simulink model "WECModel"  (R2021a)
settings: Solver=VariableStepAuto  StartTime=0.0  StopTime=30  RelTol=1e-3
undefined symbols (not defined in the file): A_c, alpha, beta, c33, delta, f_excitation_imaginary, f_excitation_real, g, gamma, H_s, k, m, m33, omega, rho
settings Model: Creator=Flamehog  LastModifiedBy=Flamehog

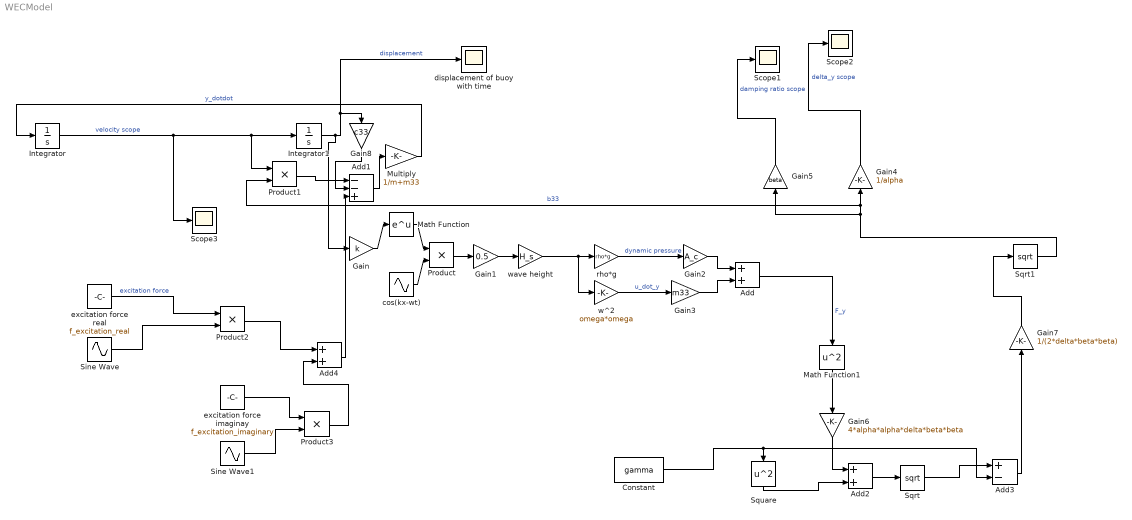
== system WECModel ==
  Add : Sum
  Add1 : Sum  Inputs=--+
  Add2 : Sum
  Add3 : Sum  Inputs=+-
  Add4 : Sum
  Constant : Constant  Value=gamma
  Gain : Gain  Gain=k
  Gain1 : Gain  Gain=0.5
  Gain2 : Gain  Gain=A_c
  Gain3 : Gain  Gain=m33
  Gain4 : Gain  Gain=1/alpha
  Gain5 : Gain  Gain=beta
  Gain6 : Gain  Gain=4*alpha*alpha*delta*beta*beta
  Gain7 : Gain  Gain=1/(2*delta*beta*beta)
  Gain8 : Gain  Gain=c33
  Integrator : Integrator
  Integrator1 : Integrator
  Math Function : Math  SaturateOnIntegerOverflow=on
  Math Function1 : Math  Operator=square  SaturateOnIntegerOverflow=on
  Multiply : Gain  Gain=1/m+m33
  Product{,1..3} (4 alike) : Product
  Scope1 : Scope
  Scope2 : Scope
  Scope3 : Scope
  Sine Wave : Sin  Amplitude=-1  Frequency=omega  Phase=pi/2  SampleTime=0
  Sine Wave1 : Sin  SampleTime=0
  Sqrt : Sqrt  SaturateOnIntegerOverflow=on
  Sqrt1 : Sqrt  SaturateOnIntegerOverflow=on
  Square : Math  Operator=square  SaturateOnIntegerOverflow=on
  cos(kx-wt) : Sin  Amplitude=-1  Frequency=omega  Phase=pi/2  SampleTime=0
  displacement of buoy with time : Scope
  excitation force imaginay : Constant  Value=f_excitation_imaginary
  excitation force real : Constant  Value=f_excitation_real
  rho*g : Gain  Gain=rho*g
  w^2 : Gain  Gain=omega*omega
  wave height : Gain  Gain=H_s
  wires:
  Integrator/1 -> Integrator1/1, Product1/1, Scope3/1  "velocity scope"
  Integrator1/1 -> Gain/1, Gain8/1, displacement of buoy with time/1  "displacement"
  Product1/1 -> Add1/1
  excitation force real/1 -> Product2/1  "excitation force"
  Add1/1 -> Multiply/1
  Multiply/1 -> Integrator/1  "y_dotdot"
  Gain/1 -> Math Function/1
  Math Function/1 -> Product/1
  cos(kx-wt)/1 -> Product/2
  Product/1 -> Gain1/1
  Gain1/1 -> wave height/1
  wave height/1 -> rho*g/1, w^2/1
  w^2/1 -> Gain3/1  "u_dot_y"
  rho*g/1 -> Gain2/1  "dynamic pressure"
  Gain2/1 -> Add/1
  Gain3/1 -> Add/2
  Add/1 -> Math Function1/1  "F_y"
  Sqrt1/1 -> Product1/2, Gain4/1, Gain5/1  "b33"
  Gain4/1 -> Scope2/1  "delta_y scope"
  Gain5/1 -> Scope1/1  "damping ratio scope"
  Math Function1/1 -> Gain6/1
  Gain6/1 -> Add2/1
  Constant/1 -> Add3/2, Square/1
  Square/1 -> Add2/2
  Add2/1 -> Sqrt/1
  Sqrt/1 -> Add3/1
  Add3/1 -> Gain7/1
  Gain7/1 -> Sqrt1/1
  Sine Wave/1 -> Product2/2
  Product2/1 -> Add4/1
  Gain8/1 -> Add1/2
  excitation force imaginay/1 -> Product3/1
  Sine Wave1/1 -> Product3/2
  Product3/1 -> Add4/2
  Add4/1 -> Add1/3
